simulink model "mcb_pmsm_foc_hall_hvkit_f28069m"  (R2021b)
settings: Solver=FixedStepDiscrete  StartTime=0.0  StopTime=8  RelTol=1e-3  EnableMultiTasking=on
InitFcn:
  | mcb_pmsm_foc_hall_hvkit_f28069m_data;
values from neighbouring files (symbols this model uses):
  inverter = mcb_SetInverterParameters('BoostXL-DRV8305')    [mcb_pmsm_foc_dual_f28379d_data.m]    (also in mcb_pmsm_foc_dual_f28379d_datascript.m; mcb_pmsm_foc_f280049C_data.m; mcb_pmsm_foc_f28335_data.m = mcb_SetInverterParameters('DRV8312-C2-KIT'); mcb_pmsm_foc_hall_f28035_data.m = mcb_SetInverterParameters('DRV8312-C2-KIT'))
  PI_params = mcb.internal.SetControllerParameters(pmsm,inverter,PU_System,T_pwm,2*Ts,Ts_speed)    [mcb_pmsm_foc_dual_f28379d_data.m]    (also in mcb_pmsm_foc_dual_f28379d_datascript.m; mcb_pmsm_foc_f280049C_data.m = mcb.internal.SetControllerParameters(pmsm,inverter,PU_System; mcb_pmsm_foc_f28335_data.m = mcb.internal.SetControllerParameters(pmsm,inverter,PU_System; mcb_pmsm_foc_hall_f28035_data.m = mcb.internal.SetControllerParameters(pmsm,inverter,PU_System)
  pmsm = struct    [c28335_pmsmfoc_data.m]    (also in mcb_pmsm_foc_dual_f28379d_data.m = mcb_SetPMSMMotorParameters('Teknic2310P'); mcb_pmsm_foc_dual_f28379d_datascript.m = mcb_SetPMSMMotorParameters('Teknic2310P'); mcb_pmsm_foc_f280049C_data.m = mcb_SetPMSMMotorParameters('BLY171D'); mcb_pmsm_foc_f28335_data.m = mcb_SetPMSMMotorParameters('BLY171D'))
  target = mcb_SetProcessorDetails('F28379D',PWM_frequency)    [mcb_pmsm_foc_dual_f28379d_data.m]    (also in mcb_pmsm_foc_dual_f28379d_datascript.m; mcb_pmsm_foc_f280049C_data.m = mcb_SetProcessorDetails('F280049C',PWM_frequency); mcb_pmsm_foc_f28335_data.m = mcb_SetProcessorDetails('F28335',PWM_frequency); mcb_pmsm_foc_hall_f28035_data.m = mcb_SetProcessorDetails('F28035',PWM_frequency))
  Ts = 5e-8    (= 5e-08)    [DCDC_Buck_Param.m]    (also in mcb_c2000_open_loop_control_data.m = T_pwm; mcb_c2000_pmsm_offset_data.m = T_pwm; mcb_pmsm_foc_dual_f28379d_data.m = 5e-05; mcb_pmsm_foc_dual_f28379d_datascript.m = 5e-05)
  Ts_motor = T_pwm/2    (= 2.5e-05)    [mcb_pmsm_foc_dual_f28379d_data.m]    (also in mcb_pmsm_foc_dual_f28379d_datascript.m; mcb_pmsm_foc_f280049C_data.m; mcb_pmsm_foc_f28335_data.m; mcb_pmsm_foc_hall_f28035_data.m)
  Ts_simulink = T_pwm/2    (= 2.5e-05)    [mcb_pmsm_foc_dual_f28379d_data.m]    (also in mcb_pmsm_foc_dual_f28379d_datascript.m; mcb_pmsm_foc_f280049C_data.m; mcb_pmsm_foc_f28335_data.m; mcb_pmsm_foc_hall_f28035_data.m)
undefined symbols (not defined in the file or in its folder): Down, GPTRIP1SEL, GPTRIP2SEL, TZ1, TZ2, Up
libraries: simulink x10, mcbpositiondecoderlib x7, idelinklib_common x5, c2802xlib x5, c280xlib x3, c2806xlib x3, svdutilitieslib x2, mcbcontrolslib x2, demo_controls x1, hall_sensor_lib x1, c2000lib x1, mcbplantlib x1
(part 2 of 2)

== system mcb_pmsm_foc_hall_hvkit_f28069m/Embedded Processor/Hall Algorithm/Input Scaling/Read_Sensor (codegen) ==
  Iab_meas_ADC : Inport  OutDataTypeStr=uint16
  Pos_Sim : Inport  Port=2  OutDataTypeStr=uint16
  Calculate Position from Hall : Subsystem
  Constant : Constant  OutDataTypeStr=boolean
  Convert ADC value to PU : Subsystem
  Terminator1 : Terminator
  Iab_Meas_PU : Outport  VectorParamsAs1DForOutWhenUnconnected=off
  Pos_PU : Outport  Port=2  VectorParamsAs1DForOutWhenUnconnected=off
  Speed_PU : Outport  Port=3  VectorParamsAs1DForOutWhenUnconnected=off
  EnClosedLoop : Outport  Port=4  VectorParamsAs1DForOutWhenUnconnected=off
  wires:
  Calculate Position from Hall/1(Pos_PU) -> Pos_PU/1
  Iab_meas_ADC/1 -> Convert ADC value to PU/1(Iab_meas_ADC)
  Convert ADC value to PU/1(Iab_meas_PU) -> Iab_Meas_PU/1
  Pos_Sim/1 -> Terminator1/1
  Calculate Position from Hall/2(Speed_PU) -> Speed_PU/1
  Constant/1 -> EnClosedLoop/1

== system mcb_pmsm_foc_hall_hvkit_f28069m/Embedded Processor/Hall Algorithm/Input Scaling/Read_Sensor (sim) ==
  Iab_meas_ADC : Inport
  Pos_Sim : Inport  Port=2
  Constant : Constant  OutDataTypeStr=boolean
  Convert ADC value to PU : Subsystem
  Subsystem : Subsystem
  Iab_Meas_PU : Outport  VectorParamsAs1DForOutWhenUnconnected=off
  Pos_PU : Outport  Port=2  VectorParamsAs1DForOutWhenUnconnected=off
  Speed_PU : Outport  Port=3  VectorParamsAs1DForOutWhenUnconnected=off
  EnClosedLoop : Outport  Port=4  VectorParamsAs1DForOutWhenUnconnected=off
  wires:
  Iab_meas_ADC/1 -> Convert ADC value to PU/1(Iab_meas_ADC)
  Convert ADC value to PU/1(Iab_meas_PU) -> Iab_Meas_PU/1
  Pos_Sim/1 -> Subsystem/1(Pos_Sim)
  Subsystem/1(Theta) -> Pos_PU/1
  Subsystem/2(Speed) -> Speed_PU/1
  Constant/1 -> EnClosedLoop/1

== system mcb_pmsm_foc_hall_hvkit_f28069m/Embedded Processor/Hall Sensor A/Capture Event Selection/Output 0 ==
  Action Port : ActionPort  ActionPortLabel=if((u1 == 5 | u1 == 3))
  Constant : Constant  OutDataTypeStr=boolean
  Out1 : Outport
  wires:
  Constant/1 -> Out1/1

== system mcb_pmsm_foc_hall_hvkit_f28069m/Embedded Processor/Hall Sensor A/Capture Event Selection/Output 1 ==
  Action Port : ActionPort  ActionPortLabel=else
  Constant : Constant  Value=0  OutDataTypeStr=boolean
  Out1 : Outport
  wires:
  Constant/1 -> Out1/1

== system mcb_pmsm_foc_hall_hvkit_f28069m/Embedded Processor/Hall Sensor A/Ecap Sensor/Code generation ==
  eCAP : c280xlib/eCAP  operatingMode=eCAP  selectCAPx=eCAP1  offsetValue=0  counterSynIn=off  enableCounter=off  syncOutput=Disabled  sampleTime=-1  eventPrescaler=0  selectMode=Continuous  enableOneShot=off  stopValue=Capture Event 2  resetEv1Ts=on  ev1Polarity=Rising Edge  resetEv2Ts=on  ev2Polarity=Falling Edge  resetEv3Ts=off  ev3Polarity=Rising Edge  resetEv4Ts=off  ev4Polarity=Rising Edge  tSCntrDataType=uint32  capEvFlag=off  capFlagDataType=uint16  overFlowFlag=off  overFlowFlagDataType=uint16  periodUnit=Seconds  periodSource=Specify via dialog  waveformPeriod=0.001  dutyUnit=Percentages  dutySource=Specify via dialog  dutyCycle=50  outputPolarity=Active High  enableCEVT1Int=on  enableCEVT2Int=on  enableCEVT3Int=off  enableCEVT4Int=off  enableCTROVFInt=on  enablePRDInt=off  enableCMPInt=off
      settings: SourceProductBaseCode=TIC2000
  eCAP_Out : Outport
  wires:
  eCAP/1 -> eCAP_Out/1

== system mcb_pmsm_foc_hall_hvkit_f28069m/Embedded Processor/Hall Sensor A/Ecap Sensor/Simulation ==
  Ground : Ground
  Ground1 : Ground
  Mux : Mux  Inputs=2
  eCAP_Out : Outport
  wires:
  Ground1/1 -> Mux/2
  Mux/1 -> eCAP_Out/1
  Ground/1 -> Mux/1

== system mcb_pmsm_foc_hall_hvkit_f28069m/Embedded Processor/Hall Sensor A/Hall Reading/CodeGen ==
  Data Type Conversion : DataTypeConversion  OutDataTypeStr=uint32  ConvertRealWorld=Stored Integer (SI)
  Read Halls : hall_sensor_lib/Read_halls  sample_time=-1
      settings: SourceProductBaseCode=TIC2000
  Out1 : Outport
  wires:
  Read Halls/1 -> Data Type Conversion/1
  Data Type Conversion/1 -> Out1/1

== system mcb_pmsm_foc_hall_hvkit_f28069m/Embedded Processor/Hall Sensor A/Hall Reading/Sim ==
  Data Type Conversion : DataTypeConversion  OutDataTypeStr=uint32  ConvertRealWorld=Stored Integer (SI)
  Ground : Ground
  Out1 : Outport
  wires:
  Data Type Conversion/1 -> Out1/1
  Ground/1 -> Data Type Conversion/1

== system mcb_pmsm_foc_hall_hvkit_f28069m/Embedded Processor/Hall Sensor B/Capture Event Selection/Output 0 ==
  Action Port : ActionPort  ActionPortLabel=else
  Constant : Constant  Value=0  OutDataTypeStr=boolean
  Out1 : Outport
  wires:
  Constant/1 -> Out1/1

== system mcb_pmsm_foc_hall_hvkit_f28069m/Embedded Processor/Hall Sensor B/Capture Event Selection/Output 1 ==
  Action Port : ActionPort  ActionPortLabel=if((u1 == 3 | u1 == 6))
  Constant : Constant  OutDataTypeStr=boolean
  Out1 : Outport
  wires:
  Constant/1 -> Out1/1

== system mcb_pmsm_foc_hall_hvkit_f28069m/Embedded Processor/Hall Sensor C/Capture Event Selection/Output 0 ==
  Action Port : ActionPort  ActionPortLabel=else
  Constant : Constant  Value=0  OutDataTypeStr=boolean
  Out1 : Outport
  wires:
  Constant/1 -> Out1/1

== system mcb_pmsm_foc_hall_hvkit_f28069m/Embedded Processor/Hall Sensor C/Capture Event Selection/Output 1 ==
  Action Port : ActionPort  ActionPortLabel=if((u1 == 5 | u1 == 6))
  Constant : Constant  OutDataTypeStr=boolean
  Out1 : Outport
  wires:
  Constant/1 -> Out1/1

== system mcb_pmsm_foc_hall_hvkit_f28069m/Embedded Processor/Hardware Init/Offset Calculation/Code Generation ==
  DRV Enable : Subsystem  Priority=1
  Default ADC Offset : Subsystem  Priority=1001  TreatAsAtomicUnit=on

== system mcb_pmsm_foc_hall_hvkit_f28069m/Embedded Processor/Hardware Init/Offset Calculation/Simulation ==

== system mcb_pmsm_foc_hall_hvkit_f28069m/Embedded Processor/Heartbeat LED/LED BLINK/Code generation ==
  note: Heartbeat LED 1HZ
  In1 : Inport
  Digital Output1 : c2806xlib/Digital Output  GPIO_Number=GPIO24~GPIO31  GPIO_Bit0=off  GPIO_BIT0_Toggle=off  GPIO_Bit1=off  GPIO_BIT1_Toggle=off  GPIO_Bit2=off  GPIO_BIT2_Toggle=off  GPIO_Bit3=off  GPIO_BIT3_Toggle=off  GPIO_Bit4=off  GPIO_BIT4_Toggle=off  GPIO_Bit5=off  GPIO_BIT5_Toggle=off  GPIO_Bit6=off  GPIO_BIT6_Toggle=off  GPIO_Bit7=on  GPIO_BIT7_Toggle=on
      settings: SourceProductBaseCode=TIC2000
  wires:
  In1/1 -> Digital Output1/1

== system mcb_pmsm_foc_hall_hvkit_f28069m/Embedded Processor/Heartbeat LED/LED BLINK/Simulation ==
  In1 : Inport
  Simulation_Terminator : Terminator
  wires:
  In1/1 -> Simulation_Terminator/1

== system mcb_pmsm_foc_hall_hvkit_f28069m/Inverter and Motor - Plant Model/Plant Model/Simulation/Average Inverter ==
  Duty_abc : Inport
  Average-Value Inverter : mcbplantlib/Average-Value Inverter
  Constant2 : Constant  Value=inverter.V_dc  OutDataTypeStr=single  SampleTime=-1
  Data Type Conversion1 : DataTypeConversion  OutDataTypeStr=single  RndMeth=Simplest
  Rate Transition3 : RateTransition  Integrity=off  OutPortSampleTime=Ts_inverter
  Vabc : Outport  VectorParamsAs1DForOutWhenUnconnected=off
  wires:
  Data Type Conversion1/1 -> Rate Transition3/1
  Duty_abc/1 -> Data Type Conversion1/1
  Rate Transition3/1 -> Average-Value Inverter/1
  Constant2/1 -> Average-Value Inverter/2
  Average-Value Inverter/1 -> Vabc/1

== system mcb_pmsm_foc_hall_hvkit_f28069m/Inverter and Motor - Plant Model/Plant Model/Simulation/Load_Profile (Torque) ==
  Data Type Conversion : DataTypeConversion  OutDataTypeStr=single
  IIR Filter : mcbcontrolslib/IIR Filter  VariantControl=Low Pass Filter  VariantSelect=Low-pass  Filter_constant=0.01  advancedSettings=off  Ts=50e-6  cutOff_freq=32.1525
      settings: SourceProductBaseCode=MT
  T_load : Step  Time=1.5  Before=0.05*pmsm.T_rated  After=0.5*pmsm.T_rated  SampleTime=Ts_simulink
  Load_Trq : Outport  VectorParamsAs1DForOutWhenUnconnected=off
  wires:
  T_load/1 -> Data Type Conversion/1
  Data Type Conversion/1 -> IIR Filter/1
  IIR Filter/1 -> Load_Trq/1

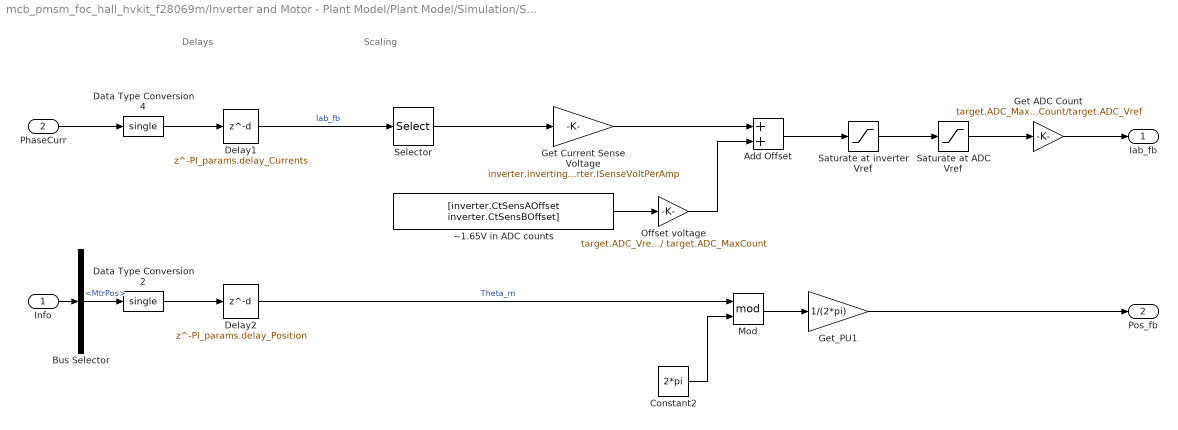
== system mcb_pmsm_foc_hall_hvkit_f28069m/Inverter and Motor - Plant Model/Plant Model/Simulation/Sensor_Measurements ==
  note: Scaling
  note: Delays
  Info : Inport
  PhaseCurr : Inport  Port=2
  Add Offset : Sum  RndMeth=Simplest
  Bus Selector : BusSelector  OutputSignals=MtrPos
  Constant2 : Constant  Value=2*pi  OutDataTypeStr=single  SampleTime=-1
  Data Type Conversion2 : DataTypeConversion  OutDataTypeStr=single  RndMeth=Simplest
  Data Type Conversion4 : DataTypeConversion  OutDataTypeStr=single  RndMeth=Simplest
  Delay1 : Delay  DelayLength=PI_params.delay_Currents
  Delay2 : Delay  DelayLength=PI_params.delay_Position
  Get ADC Count : Gain  Gain=target.ADC_MaxCount/target.ADC_Vref  OutMin=0  OutMax=target.ADC_MaxCount  OutDataTypeStr=uint16  RndMeth=Simplest
  Get Current Sense Voltage : Gain  Gain=inverter.invertingAmp * inverter.ISenseVoltPerAmp  RndMeth=Simplest  OutDataTypeStr=Inherit: Same as input
  Get_PU1 : Gain  Gain=1/(2*pi)  OutDataTypeStr=dataType  RndMeth=Simplest
  Mod : Math  Operator=mod  SaturateOnIntegerOverflow=on
  Offset voltage : Gain  Gain=target.ADC_Vref / target.ADC_MaxCount  RndMeth=Simplest
  Saturate at ADC Vref : Saturate  UpperLimit=target.ADC_Vref  LowerLimit=0
  Saturate at inverter Vref : Saturate  UpperLimit=inverter.ISenseVref  LowerLimit=0
  Selector : Selector  InputPortWidth=3  IndexOptions=Index vector (dialog)  Indices=[1 2]  OutputSizes=1
  ~1.65V in ADC counts : Constant  Value=[inverter.CtSensAOffset inverter.CtSensBOffset]  OutDataTypeStr=uint16  SampleTime=-1
  Iab_fb : Outport  VectorParamsAs1DForOutWhenUnconnected=off
  Pos_fb : Outport  Port=2  VectorParamsAs1DForOutWhenUnconnected=off
  wires:
  Delay1/1 -> Selector/1  "Iab_fb"
  Data Type Conversion4/1 -> Delay1/1
  PhaseCurr/1 -> Data Type Conversion4/1
  Info/1 -> Bus Selector/1
  Bus Selector/1 -> Data Type Conversion2/1  "<MtrPos>"
  Data Type Conversion2/1 -> Delay2/1
  Delay2/1 -> Mod/1  "Theta_m"
  Get_PU1/1 -> Pos_fb/1
  Mod/1 -> Get_PU1/1
  Constant2/1 -> Mod/2
  Get ADC Count/1 -> Iab_fb/1
  Selector/1 -> Get Current Sense Voltage/1
  Add Offset/1 -> Saturate at inverter Vref/1
  Get Current Sense Voltage/1 -> Add Offset/1
  ~1.65V in ADC counts/1 -> Offset voltage/1
  Saturate at inverter Vref/1 -> Saturate at ADC Vref/1
  Offset voltage/1 -> Add Offset/2
  Saturate at ADC Vref/1 -> Get ADC Count/1

== system mcb_pmsm_foc_hall_hvkit_f28069m/Embedded Processor/Hall Algorithm/Input Scaling/Read_Sensor (codegen)/Calculate Position from Hall ==
  note: Note: The glitch filter rejects lower values of the speed count input, which resutls in motor speed greater than 10 times Base speed
  Atomic Hall Reading : Subsystem  TreatAsAtomicUnit=on
  Data Store Write2 : DataStoreWrite  Priority=2  DataStoreName=HallStateChangeFlag  IndexOptions=Index vector (dialog)  Indices=1  OutputSizes=1
  Glitch Filter : simulink/Logic and Bit Operations/Compare To Constant  relop=>=  const=target.CPU_frequency * 60 / (pmsm.N_base * 10 * 2 * pmsm.p)  OutDataTypeStr=boolean
  Hall Speed and Position : mcbpositiondecoderlib/Hall Speed and Position  blkExecutionType=Speed and position  CounterSize=32 bits  ClkFreq=target.CPU_frequency  BlkSampleTime=Ts  PolePairs=pmsm.p  MinSpeed=20  HallInterruptConfig=Every 180 Degrees  SpeedUnit=Per unit  PerUnitSpeed=PU_System.N_base  SpeedDataType=dataType  hallSequence=ABC  Sequence=[5,4,6,2,3,1]  EnableSecondOrder=1st Order  PositionUnit=Per unit  PositionDataType=dataType
      settings: SourceProductBaseCode=MT
  Mechanical to Electrical Position : mcbpositiondecoderlib/Mechanical to Electrical Position  NrPP=1  selectedRange=Per unit  MechOfstInputType=Specify via dialog  mechOffsetIn=pmsm.PositionOffset  maxAngleIn=1  InputDataType=dataType  VariantSelect=floating-point
      settings: SourceProductBaseCode=MT
  Subsystem : Subsystem
  Pos_PU : Outport  InitialOutput=0  VectorParamsAs1DForOutWhenUnconnected=off
  Speed_PU : Outport  Port=2  InitialOutput=0  VectorParamsAs1DForOutWhenUnconnected=off
  wires:
  Hall Speed and Position/3 -> Data Store Write2/1
  Hall Speed and Position/1 -> Mechanical to Electrical Position/1
  Mechanical to Electrical Position/1 -> Pos_PU/1
  Hall Speed and Position/2 -> Speed_PU/1
  Atomic Hall Reading/1(HallState) -> Hall Speed and Position/1
  Atomic Hall Reading/2(Count) -> Hall Speed and Position/2
  Atomic Hall Reading/4(Dir) -> Hall Speed and Position/4
  Atomic Hall Reading/5(SpeedValidity) -> Hall Speed and Position/5
  Atomic Hall Reading/6(Hallchange) -> Hall Speed and Position/6
  Glitch Filter/1 -> Subsystem/Enable
  Atomic Hall Reading/3(SpeedCount) -> Glitch Filter/1, Subsystem/1(Input)
  Subsystem/1(Output) -> Hall Speed and Position/3

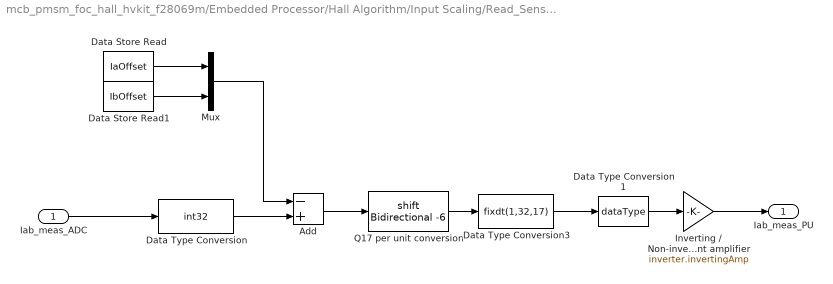
== system mcb_pmsm_foc_hall_hvkit_f28069m/Embedded Processor/Hall Algorithm/Input Scaling/Read_Sensor (codegen)/Convert ADC value to PU ==
  Iab_meas_ADC : Inport
  Add : Sum  Inputs=-+
  Data Store Read : DataStoreRead  DataStoreName=IaOffset  IndexOptions=Index vector (dialog)  Indices=1  OutputSizes=1
  Data Store Read1 : DataStoreRead  DataStoreName=IbOffset  IndexOptions=Index vector (dialog)  Indices=1  OutputSizes=1
  Data Type Conversion : DataTypeConversion  OutDataTypeStr=int32  ConvertRealWorld=Stored Integer (SI)
  Data Type Conversion1 : DataTypeConversion  OutDataTypeStr=dataType
  Data Type Conversion3 : DataTypeConversion  OutDataTypeStr=fixdt(1,32,17)  ConvertRealWorld=Stored Integer (SI)  RndMeth=Simplest
  Inverting / Non-inverting Current measurement amplifier : Gain  Gain=inverter.invertingAmp  RndMeth=Simplest  OutDataTypeStr=Inherit: Same as input
  Mux : Mux  Inputs=2
  Q17 per unit conversion : ArithShift  BitShiftNumber=-6
  Iab_meas_PU : Outport  InitialOutput=0  VectorParamsAs1DForOutWhenUnconnected=off
  wires:
  Data Type Conversion3/1 -> Data Type Conversion1/1
  Add/1 -> Q17 per unit conversion/1
  Data Type Conversion/1 -> Add/2
  Iab_meas_ADC/1 -> Data Type Conversion/1
  Q17 per unit conversion/1 -> Data Type Conversion3/1
  Data Store Read1/1 -> Mux/2
  Data Store Read/1 -> Mux/1
  Mux/1 -> Add/1
  Data Type Conversion1/1 -> Inverting / Non-inverting Current measurement amplifier/1
  Inverting / Non-inverting Current measurement amplifier/1 -> Iab_meas_PU/1

== system mcb_pmsm_foc_hall_hvkit_f28069m/Embedded Processor/Hall Algorithm/Input Scaling/Read_Sensor (sim)/Convert ADC value to PU ==
  Iab_meas_ADC : Inport
  0A in ADC counts : Constant  Value=[inverter.CtSensAOffset inverter.CtSensBOffset]  OutDataTypeStr=int32  SampleTime=-1
  Add : Sum  Inputs=-+
  Data Type Conversion : DataTypeConversion  OutDataTypeStr=int32  ConvertRealWorld=Stored Integer (SI)
  Data Type Conversion1 : DataTypeConversion  OutDataTypeStr=dataType
  Data Type Conversion3 : DataTypeConversion  OutDataTypeStr=fixdt(1,32,17)  ConvertRealWorld=Stored Integer (SI)  RndMeth=Simplest
  Inverting / Non-inverting Current measurement amplifier : Gain  Gain=inverter.invertingAmp  RndMeth=Simplest  OutDataTypeStr=Inherit: Same as input
  Q17 per unit conversion : ArithShift  BitShiftNumber=-6
  Iab_meas_PU : Outport  InitialOutput=0  VectorParamsAs1DForOutWhenUnconnected=off
  wires:
  Data Type Conversion3/1 -> Data Type Conversion1/1
  Add/1 -> Q17 per unit conversion/1
  Data Type Conversion/1 -> Add/2
  Iab_meas_ADC/1 -> Data Type Conversion/1
  0A in ADC counts/1 -> Add/1
  Q17 per unit conversion/1 -> Data Type Conversion3/1
  Data Type Conversion1/1 -> Inverting / Non-inverting Current measurement amplifier/1
  Inverting / Non-inverting Current measurement amplifier/1 -> Iab_meas_PU/1

== system mcb_pmsm_foc_hall_hvkit_f28069m/Embedded Processor/Hall Algorithm/Input Scaling/Read_Sensor (sim)/Subsystem ==
  Pos_Sim : Inport
  IIR Filter : mcbcontrolslib/IIR Filter  VariantControl=Low Pass Filter  VariantSelect=Low-pass  Filter_constant=0.01  advancedSettings=off  Ts=50e-6  cutOff_freq=32.1525
      settings: SourceProductBaseCode=MT
  Mechanical to Electrical Position : mcbpositiondecoderlib/Mechanical to Electrical Position  NrPP=pmsm.p  selectedRange=Per unit  MechOfstInputType=Specify via dialog  mechOffsetIn=0  maxAngleIn=1  InputDataType=dataType  VariantSelect=floating-point
      settings: SourceProductBaseCode=MT
  Speed Measurement : mcbpositiondecoderlib/Speed Measurement  PositionUnit=Per unit  PositionScalingDatatype=uint32  SpeedCalculationMode=Time interval for speed calculation  SampleTimeAsync=Ts  MaximumApplicationSpeed=6000  SpeedResolution=5e-6  DelayLength=10  MaximumMeasurableSpeed=59999  MeasurableSpeedResolution=2.794e-05  SpeedUnit=Per unit based on dialog  PerUnitSpeed=PU_System.N_base  SpeedDataType=dataType
      settings: SourceProductBaseCode=MT
  Theta : Outport
  Speed : Outport  Port=2
  wires:
  Mechanical to Electrical Position/1 -> Theta/1
  IIR Filter/1 -> Speed/1
  Speed Measurement/1 -> IIR Filter/1
  Pos_Sim/1 -> Speed Measurement/1, Mechanical to Electrical Position/1

== system mcb_pmsm_foc_hall_hvkit_f28069m/Embedded Processor/Hardware Init/Offset Calculation/Code Generation/DRV Enable ==
  note: Enable PWM output
  Digital Output1 : c2806xlib/Digital Output  GPIO_Number=GPIO8~GPIO15  GPIO_Bit0=off  GPIO_BIT0_Toggle=off  GPIO_Bit1=off  GPIO_BIT1_Toggle=off  GPIO_Bit2=off  GPIO_BIT2_Toggle=off  GPIO_Bit3=off  GPIO_BIT3_Toggle=off  GPIO_Bit4=off  GPIO_BIT4_Toggle=off  GPIO_Bit5=off  GPIO_BIT5_Toggle=off  GPIO_Bit6=off  GPIO_BIT6_Toggle=off  GPIO_Bit7=on  GPIO_BIT7_Toggle=off
      settings: SourceProductBaseCode=TIC2000
  INV Enable : Constant  Value=0  OutDataTypeStr=uint16
  wires:
  INV Enable/1 -> Digital Output1/1

== system mcb_pmsm_foc_hall_hvkit_f28069m/Embedded Processor/Hardware Init/Offset Calculation/Code Generation/Default ADC Offset ==
  Constant : Constant  Value=inverter.CtSensAOffset  OutDataTypeStr=Inherit: Inherit via back propagation
  Constant1 : Constant  Value=inverter.CtSensBOffset  OutDataTypeStr=Inherit: Inherit via back propagation
  Data Store Write1 : DataStoreWrite  DataStoreName=IaOffset  IndexOptions=Index vector (dialog)  Indices=1  OutputSizes=1
  Data Store Write2 : DataStoreWrite  DataStoreName=IbOffset  IndexOptions=Index vector (dialog)  Indices=1  OutputSizes=1
  wires:
  Constant/1 -> Data Store Write1/1
  Constant1/1 -> Data Store Write2/1

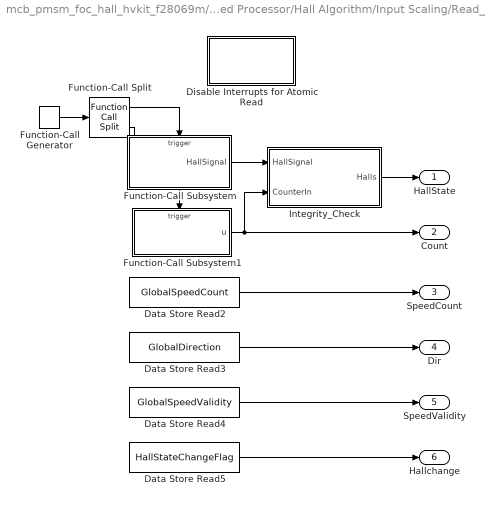
== system mcb_pmsm_foc_hall_hvkit_f28069m/Embedded Processor/Hall Algorithm/Input Scaling/Read_Sensor (codegen)/Calculate Position from Hall/Atomic Hall Reading ==
  Data Store Read2 : DataStoreRead  DataStoreName=GlobalSpeedCount  IndexOptions=Index vector (dialog)  Indices=1  OutputSizes=1
  Data Store Read3 : DataStoreRead  DataStoreName=GlobalDirection  IndexOptions=Index vector (dialog)  Indices=1  OutputSizes=1
  Data Store Read4 : DataStoreRead  DataStoreName=GlobalSpeedValidity  IndexOptions=Index vector (dialog)  Indices=1  OutputSizes=1
  Data Store Read5 : DataStoreRead  Priority=1  DataStoreName=HallStateChangeFlag  IndexOptions=Index vector (dialog)  Indices=1  OutputSizes=1
  Disable Interrupts for Atomic Read : Subsystem  mask(System Outputs){ShowInLibBrowser=0}
      mask prompts: ShowInLibBrowser "Simulink:masks:CustCodeMaskParam1_MP"
      settings: CopyFcn=cccopyfcn(gcb)  OpenFcn=ccopenfcn('System Outputs Function')
      mask Help: eval('feval(''rtwprivate'',''rtwhelpview'',''rtw_sys_outputs_block'')');
      mask Display: disp('System\nOutputs');
  Function-Call Generator : simulink/Ports & Subsystems/Function-Call Generator  sample_time=-1  numberOfIterations=1  DisallowWideOutput=off
  Function-Call Split : FunctionCallSplit  NumOutputPorts=2  OutputPortLayout=default
  Function-Call Subsystem : Subsystem  TreatAsAtomicUnit=on
  Function-Call Subsystem1 : Subsystem  TreatAsAtomicUnit=on
  Integrity_Check : Subsystem
  HallState : Outport
  Count : Outport  Port=2
  SpeedCount : Outport  Port=3
  Dir : Outport  Port=4
  SpeedValidity : Outport  Port=5
  Hallchange : Outport  Port=6
  wires:
  Data Store Read4/1 -> SpeedValidity/1
  Data Store Read5/1 -> Hallchange/1
  Data Store Read2/1 -> SpeedCount/1
  Data Store Read3/1 -> Dir/1
  Function-Call Split/1 -> Function-Call Subsystem/Trigger
  Integrity_Check/1(Halls) -> HallState/1
  Function-Call Split/2 -> Function-Call Subsystem1/Trigger
  Function-Call Generator/1 -> Function-Call Split/1
  Function-Call Subsystem/1(HallSignal) -> Integrity_Check/1(HallSignal)
  Function-Call Subsystem1/1(u) -> Count/1, Integrity_Check/2(CounterIn)

== system mcb_pmsm_foc_hall_hvkit_f28069m/Embedded Processor/Hall Algorithm/Input Scaling/Read_Sensor (codegen)/Calculate Position from Hall/Subsystem ==
  Input : Inport
  Enable : EnablePort
  Output : Outport
  wires:
  Input/1 -> Output/1

== system mcb_pmsm_foc_hall_hvkit_f28069m/Embedded Processor/Hall Algorithm/Input Scaling/Read_Sensor (codegen)/Calculate Position from Hall/Atomic Hall Reading/Disable Interrupts for Atomic Read ==

== system mcb_pmsm_foc_hall_hvkit_f28069m/Embedded Processor/Hall Algorithm/Input Scaling/Read_Sensor (codegen)/Calculate Position from Hall/Atomic Hall Reading/Function-Call Subsystem ==
  function : TriggerPort  TriggerType=function-call  VariantControl=Variant
  Bitwise AND : simulink/Logic and Bit Operations/Bitwise Operator  logicop=AND  UseBitMask=on  BitMask=hex2dec('07000000')  BitMaskRealWorld=Stored Integer
  Data Type Conversion : DataTypeConversion  OutDataTypeStr=uint32  ConvertRealWorld=Stored Integer (SI)
  Memory Copy3 : svdutilitieslib/Memory Copy  copyFrom=Specified source code symbol  copyFromAddressSource=Specify via dialog  copyFromAddress=hex2dec('00001000')  copyFromSrcCode=&GpioDataRegs.GPADAT.all  dataTypeFrom=uint32  dataDimensionFrom=1  useOffsetFrom=off  offsetFromSrc=Specify via dialog  offsetFrom=0  strideFrom=1  copyTo=Output port  copyToAddressSource=Specify via dialog  copyToAddress=hex2dec('00002000')  copyToSrcCode=myVariableDst  dataTypeTo=uint32  useOffsetTo=off  offsetToSrc=Specify via dialog  offsetTo=0  strideTo=1  sampleTime=-1  useInitValue=off  initValueSrc=Specify constant value  initValue=1  initValueSrcCode=myInitValueVariable  useAsMask=off  maskOperator=bitwise AND  useTermValue=off  termValue=1  isRealtimeEnabled=off  emitCCBeforeWrite=off  CCBeforeWrite=/* Custom Code Before Write*/  emitCCAfterWrite=off  CCAfterWrite=/* Custom Code After Write*/  useDMACopy=off  enableBlockingMode=off  blockPlatform=arduinoert
      settings: SourceProductBaseCode=ANDROID,ARDUINO,ML_ARDUINO,ECCORTEXA,ECCORTEXR,SC_BEAGLEBONE_BLUE,EC_FREEDOM_BOARD,EC_FRDM_K64F,INTEL_BLOCKSET,MICROBIT,NUCLEO,NVIDIA,PX4AUTOPILOTS,RASPPIIO,STMICRODIS,TIC2000,XILINX_BLOCKSET
  Shift Arithmetic : ArithShift  BitShiftNumber=24
  HallSignal : Outport
  wires:
  Data Type Conversion/1 -> HallSignal/1
  Shift Arithmetic/1 -> Data Type Conversion/1
  Bitwise AND/1 -> Shift Arithmetic/1
  Memory Copy3/1 -> Bitwise AND/1

== system mcb_pmsm_foc_hall_hvkit_f28069m/Embedded Processor/Hall Algorithm/Input Scaling/Read_Sensor (codegen)/Calculate Position from Hall/Atomic Hall Reading/Function-Call Subsystem1 ==
  function : TriggerPort  TriggerType=function-call  VariantControl=Variant
  Memory Copy : idelinklib_common/Memory Copy  copyFrom=Specified source code symbol  copyFromAddressSource=Specify via dialog  copyFromAddress=hex2dec('00001000')  copyFromSrcCode=&ECap1Regs.TSCTR  dataTypeFrom=uint32  dataDimensionFrom=1  useOffsetFrom=off  offsetFromSrc=Specify via dialog  offsetFrom=0  strideFrom=1  copyTo=Output port  copyToAddressSource=Specify via dialog  copyToAddress=hex2dec('00002000')  copyToSrcCode=myVariableDst  dataTypeTo=uint32  useOffsetTo=off  offsetToSrc=Specify via dialog  offsetTo=0  strideTo=1  sampleTime=-1  useInitValue=off  initValueSrc=Specify constant value  initValue=1  initValueSrcCode=myInitValueVariable  useAsMask=off  maskOperator=bitwise AND  useTermValue=off  termValue=1  isRealtimeEnabled=off  emitCCBeforeWrite=off  CCBeforeWrite=/* Custom Code Before Write*/  emitCCAfterWrite=off  CCAfterWrite=/* Custom Code After Write*/  useDMACopy=off  enableBlockingMode=off
      settings: SourceProductBaseCode=ME
  Memory Copy1 : idelinklib_common/Memory Copy  copyFrom=Specified source code symbol  copyFromAddressSource=Specify via dialog  copyFromAddress=hex2dec('00001000')  copyFromSrcCode=&ECap2Regs.TSCTR  dataTypeFrom=uint32  dataDimensionFrom=1  useOffsetFrom=off  offsetFromSrc=Specify via dialog  offsetFrom=0  strideFrom=1  copyTo=Output port  copyToAddressSource=Specify via dialog  copyToAddress=hex2dec('00002000')  copyToSrcCode=myVariableDst  dataTypeTo=uint32  useOffsetTo=off  offsetToSrc=Specify via dialog  offsetTo=0  strideTo=1  sampleTime=-1  useInitValue=off  initValueSrc=Specify constant value  initValue=1  initValueSrcCode=myInitValueVariable  useAsMask=off  maskOperator=bitwise AND  useTermValue=off  termValue=1  isRealtimeEnabled=off  emitCCBeforeWrite=off  CCBeforeWrite=/* Custom Code Before Write*/  emitCCAfterWrite=off  CCAfterWrite=/* Custom Code After Write*/  useDMACopy=off  enableBlockingMode=off
      settings: SourceProductBaseCode=ME
  Memory Copy2 : idelinklib_common/Memory Copy  copyFrom=Specified source code symbol  copyFromAddressSource=Specify via dialog  copyFromAddress=hex2dec('00001000')  copyFromSrcCode=&ECap3Regs.TSCTR  dataTypeFrom=uint32  dataDimensionFrom=1  useOffsetFrom=off  offsetFromSrc=Specify via dialog  offsetFrom=0  strideFrom=1  copyTo=Output port  copyToAddressSource=Specify via dialog  copyToAddress=hex2dec('00002000')  copyToSrcCode=myVariableDst  dataTypeTo=uint32  useOffsetTo=off  offsetToSrc=Specify via dialog  offsetTo=0  strideTo=1  sampleTime=-1  useInitValue=off  initValueSrc=Specify constant value  initValue=1  initValueSrcCode=myInitValueVariable  useAsMask=off  maskOperator=bitwise AND  useTermValue=off  termValue=1  isRealtimeEnabled=off  emitCCBeforeWrite=off  CCBeforeWrite=/* Custom Code Before Write*/  emitCCAfterWrite=off  CCAfterWrite=/* Custom Code After Write*/  useDMACopy=off  enableBlockingMode=off
      settings: SourceProductBaseCode=ME
  Min : MinMax  Inputs=3
  u : Outport
  wires:
  Memory Copy1/1 -> Min/2
  Memory Copy/1 -> Min/1
  Memory Copy2/1 -> Min/3
  Min/1 -> u/1

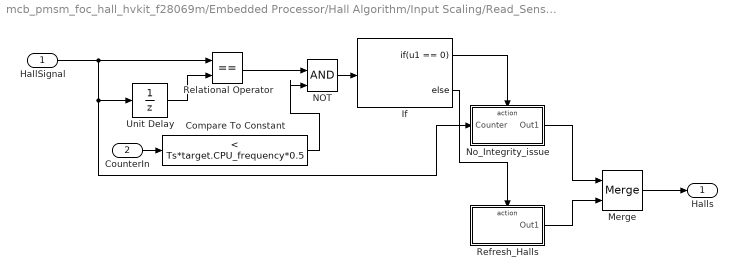
== system mcb_pmsm_foc_hall_hvkit_f28069m/Embedded Processor/Hall Algorithm/Input Scaling/Read_Sensor (codegen)/Calculate Position from Hall/Atomic Hall Reading/Integrity_Check ==
  HallSignal : Inport
  CounterIn : Inport  Port=2
  Compare To Constant : simulink/Logic and Bit Operations/Compare To Constant  relop=<  const=Ts*target.CPU_frequency*0.5  OutDataTypeStr=uint8
  If : If  IfExpression=u1 == 0
  Merge : Merge
  NOT : Logic  IconShape=distinctive  AllPortsSameDT=off  OutDataTypeStr=boolean
  No_Integrity_issue : Subsystem  TreatAsAtomicUnit=on
  Refresh_Halls : Subsystem  TreatAsAtomicUnit=on
  Relational Operator : RelationalOperator  Operator===  OutDataTypeStr=boolean  RndMeth=Simplest
  Unit Delay : UnitDelay  SampleTime=-1  HasFrameUpgradeWarning=on
  Halls : Outport
  wires:
  Refresh_Halls/1(Out1) -> Merge/2
  HallSignal/1 -> Relational Operator/1, No_Integrity_issue/1(Counter), Unit Delay/1
  If/2 -> Refresh_Halls/Action
  Merge/1 -> Halls/1
  No_Integrity_issue/1(Out1) -> Merge/1
  If/1 -> No_Integrity_issue/Action
  CounterIn/1 -> Compare To Constant/1
  Compare To Constant/1 -> NOT/2
  Relational Operator/1 -> NOT/1
  NOT/1 -> If/1
  Unit Delay/1 -> Relational Operator/2

== system mcb_pmsm_foc_hall_hvkit_f28069m/Embedded Processor/Hall Algorithm/Input Scaling/Read_Sensor (codegen)/Calculate Position from Hall/Atomic Hall Reading/Integrity_Check/No_Integrity_issue ==
  Counter : Inport
  Action Port : ActionPort  ActionPortLabel=if(u1 == 0)
  Out1 : Outport
  wires:
  Counter/1 -> Out1/1

== system mcb_pmsm_foc_hall_hvkit_f28069m/Embedded Processor/Hall Algorithm/Input Scaling/Read_Sensor (codegen)/Calculate Position from Hall/Atomic Hall Reading/Integrity_Check/Refresh_Halls ==
  Action Port : ActionPort  ActionPortLabel=else
  Bitwise AND : simulink/Logic and Bit Operations/Bitwise Operator  logicop=AND  UseBitMask=on  BitMask=hex2dec('07000000')  BitMaskRealWorld=Stored Integer
  Data Type Conversion : DataTypeConversion  OutDataTypeStr=uint32  ConvertRealWorld=Stored Integer (SI)
  Memory Copy3 : svdutilitieslib/Memory Copy  copyFrom=Specified source code symbol  copyFromAddressSource=Specify via dialog  copyFromAddress=hex2dec('00001000')  copyFromSrcCode=&GpioDataRegs.GPADAT.all  dataTypeFrom=uint32  dataDimensionFrom=1  useOffsetFrom=off  offsetFromSrc=Specify via dialog  offsetFrom=0  strideFrom=1  copyTo=Output port  copyToAddressSource=Specify via dialog  copyToAddress=hex2dec('00002000')  copyToSrcCode=myVariableDst  dataTypeTo=uint32  useOffsetTo=off  offsetToSrc=Specify via dialog  offsetTo=0  strideTo=1  sampleTime=-1  useInitValue=off  initValueSrc=Specify constant value  initValue=1  initValueSrcCode=myInitValueVariable  useAsMask=off  maskOperator=bitwise AND  useTermValue=off  termValue=1  isRealtimeEnabled=off  emitCCBeforeWrite=off  CCBeforeWrite=/* Custom Code Before Write*/  emitCCAfterWrite=off  CCAfterWrite=/* Custom Code After Write*/  useDMACopy=off  enableBlockingMode=off  blockPlatform=arduinoert
      settings: SourceProductBaseCode=ANDROID,ARDUINO,ML_ARDUINO,ECCORTEXA,ECCORTEXR,SC_BEAGLEBONE_BLUE,EC_FREEDOM_BOARD,EC_FRDM_K64F,INTEL_BLOCKSET,MICROBIT,NUCLEO,NVIDIA,PX4AUTOPILOTS,RASPPIIO,STMICRODIS,TIC2000,XILINX_BLOCKSET
  Shift Arithmetic : ArithShift  BitShiftNumber=24
  Out1 : Outport
  wires:
  Memory Copy3/1 -> Bitwise AND/1
  Bitwise AND/1 -> Shift Arithmetic/1
  Shift Arithmetic/1 -> Data Type Conversion/1
  Data Type Conversion/1 -> Out1/1
